simulink model "Solar_Batt_H2_PowerFlow_Solution"  (R2021a)
settings: Solver=ode8  StartTime=0.0  StopTime=8760  FixedStep=1  RelTol=1e-3
settings Model: Creator=pacel  LastModifiedBy=pacel

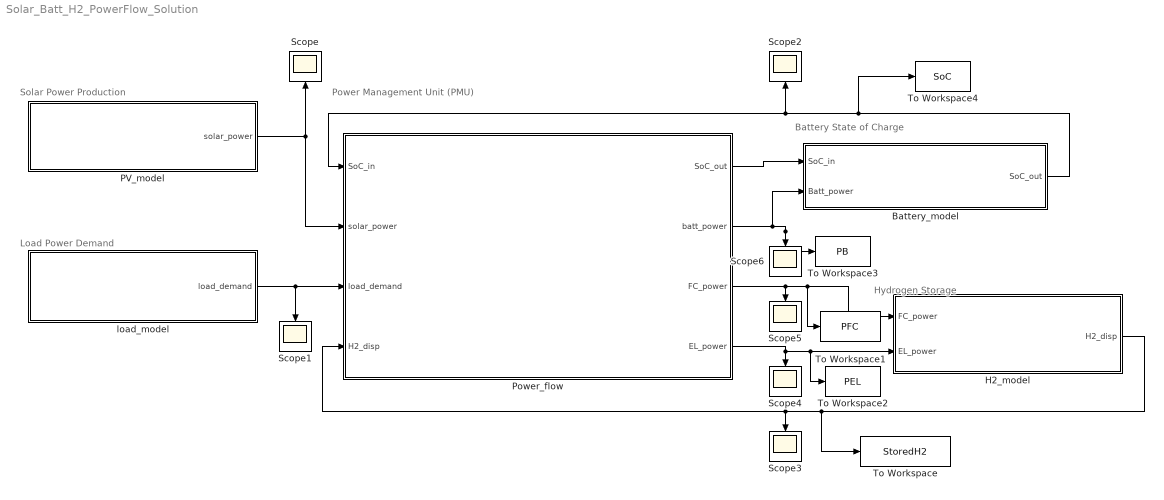
== system Solar_Batt_H2_PowerFlow_Solution ==
  note: Solar Power Production
  note: Load Power Demand
  note: Battery State of Charge
  note: Hydrogen Storage
  note: Power Management Unit (PMU)
  Battery_model : Subsystem
  H2_model : Subsystem
  PV_model : Subsystem
  Power_flow : Subsystem
  Scope{,1..6} (7 alike) : Scope
  To Workspace : ToWorkspace  VariableName=StoredH2  SaveFormat=Timeseries  SampleTime=-1
  To Workspace1 : ToWorkspace  VariableName=PFC  SaveFormat=Timeseries  SampleTime=-1
  To Workspace2 : ToWorkspace  VariableName=PEL  SaveFormat=Timeseries  SampleTime=-1
  To Workspace3 : ToWorkspace  VariableName=PB  SaveFormat=Timeseries  SampleTime=-1
  To Workspace4 : ToWorkspace  VariableName=SoC  SaveFormat=Timeseries  SampleTime=-1
  load_model : Subsystem
  wires:
  Power_flow/4(EL_power) -> Scope4/1, To Workspace2/1, H2_model/2(EL_power)
  Power_flow/3(FC_power) -> Scope5/1, H2_model/1(FC_power), To Workspace1/1
  Power_flow/2(batt_power) -> Battery_model/2(Batt_power), Scope6/1, To Workspace3/1
  H2_model/1(H2_disp) -> To Workspace/1, Power_flow/4(H2_disp), Scope3/1
  load_model/1(load_demand) -> Scope1/1, Power_flow/3(load_demand)
  PV_model/1(solar_power) -> Power_flow/2(solar_power), Scope/1
  Battery_model/1(SoC_out) -> To Workspace4/1, Scope2/1, Power_flow/1(SoC_in)
  Power_flow/1(SoC_out) -> Battery_model/1(SoC_in)

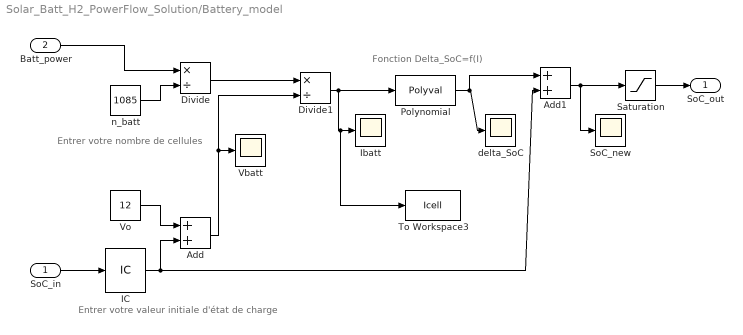
== system Solar_Batt_H2_PowerFlow_Solution/Battery_model ==
  note: Entrer votre valeur initiale d'état de charge
  note: Entrer votre nombre de cellules
  note: Fonction Delta_SoC=f(I)
  SoC_in : Inport
  Batt_power : Inport  Port=2
  Add : Sum
  Add1 : Sum
  Divide : Product  Inputs=*/
  Divide1 : Product  Inputs=*/
  IC : InitialCondition  Value=0.5
  Ibatt : Scope
  Polynomial : Polyval  Coefs=[ +8e-5, +0.0105, -0.008 ]
  Saturation : Saturate  UpperLimit=0.95  LowerLimit=0.05
  SoC_new : Scope
  To Workspace3 : ToWorkspace  VariableName=Icell  SaveFormat=Timeseries  SampleTime=-1
  Vbatt : Scope
  Vo : Constant  Value=12
  delta_SoC : Scope
  n_batt : Constant  Value=1085
  SoC_out : Outport
  wires:
  Saturation/1 -> SoC_out/1
  IC/1 -> Add1/2, Add/2
  Add1/1 -> Saturation/1, SoC_new/1
  Batt_power/1 -> Divide/1
  Add/1 -> Divide1/2, Vbatt/1
  SoC_in/1 -> IC/1
  Vo/1 -> Add/1
  Divide1/1 -> Polynomial/1, To Workspace3/1, Ibatt/1
  Divide/1 -> Divide1/1
  Polynomial/1 -> Add1/1, delta_SoC/1
  n_batt/1 -> Divide/2

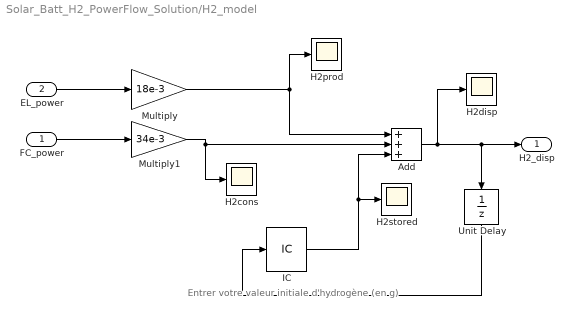
== system Solar_Batt_H2_PowerFlow_Solution/H2_model ==
  note: Entrer votre valeur initiale d'hydrogène (en g)
  FC_power : Inport
  EL_power : Inport  Port=2
  Add : Sum  Inputs=+++
  H2cons : Scope
  H2disp : Scope
  H2prod : Scope
  H2stored : Scope
  IC : InitialCondition  Value=1.2e6
  Multiply : Gain  Gain=18e-3
  Multiply1 : Gain  Gain=34e-3
  Unit Delay : UnitDelay  SampleTime=-1  HasFrameUpgradeWarning=on
  H2_disp : Outport
  wires:
  IC/1 -> Add/3, H2stored/1
  Unit Delay/1 -> IC/1
  FC_power/1 -> Multiply1/1
  EL_power/1 -> Multiply/1
  Multiply/1 -> Add/1, H2prod/1
  Multiply1/1 -> H2cons/1, Add/2
  Add/1 -> Unit Delay/1, H2_disp/1, H2disp/1

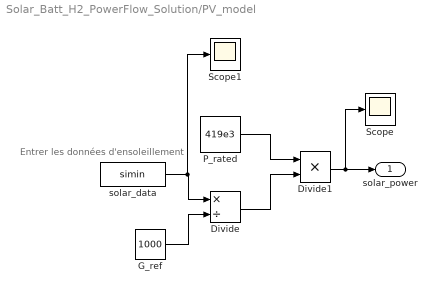
== system Solar_Batt_H2_PowerFlow_Solution/PV_model ==
  note: Entrer les données d'ensoleillement
  Divide : Product  Inputs=*/
  Divide1 : Product  Inputs=**
  G_ref : Constant  Value=1000
  P_rated : Constant  Value=419e3
  Scope : Scope
  Scope1 : Scope
  solar_data : FromWorkspace  VariableName=simin  OutDataTypeStr=double  SampleTime=1
  solar_power : Outport
  wires:
  Divide/1 -> Divide1/2
  P_rated/1 -> Divide1/1
  solar_data/1 -> Scope1/1, Divide/1
  Divide1/1 -> solar_power/1, Scope/1
  G_ref/1 -> Divide/2

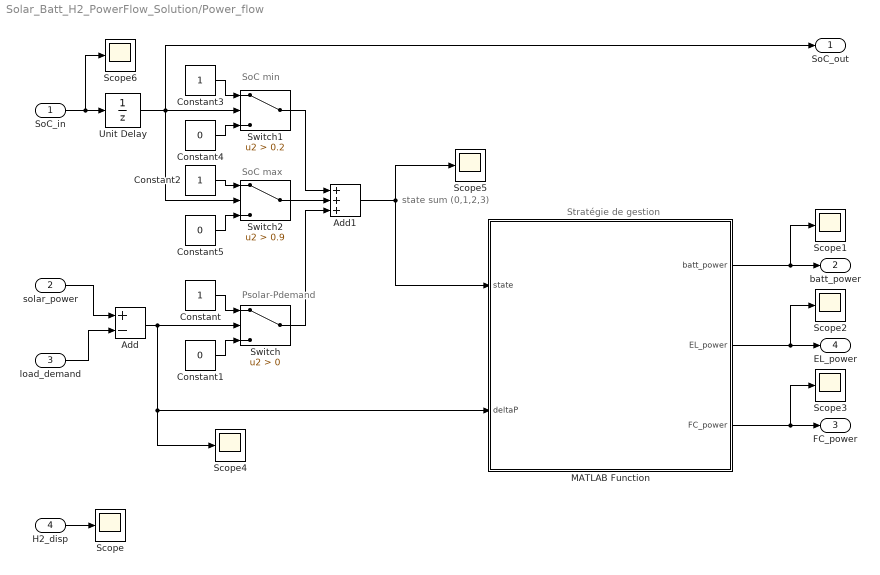
== system Solar_Batt_H2_PowerFlow_Solution/Power_flow ==
  note: SoC min
  note: SoC max
  note: Psolar-Pdemand
  note: Stratégie de gestion
  note: state sum (0,1,2,3)
  SoC_in : Inport
  solar_power : Inport  Port=2
  load_demand : Inport  Port=3
  H2_disp : Inport  Port=4
  Add : Sum  Inputs=+-
  Add1 : Sum  Inputs=+++
  Constant : Constant
  Constant1 : Constant  Value=0
  Constant2 : Constant
  Constant3 : Constant
  Constant4 : Constant  Value=0
  Constant5 : Constant  Value=0
  MATLAB Function : MATLAB Function  TreatAsAtomicUnit=on
  Scope{,1..6} (7 alike) : Scope
  Switch : Switch  Criteria=u2 > Threshold
  Switch1 : Switch  Criteria=u2 > Threshold  Threshold=0.2
  Switch2 : Switch  Criteria=u2 > Threshold  Threshold=0.9
  Unit Delay : UnitDelay  SampleTime=-1  HasFrameUpgradeWarning=on
  SoC_out : Outport
  batt_power : Outport  Port=2
  FC_power : Outport  Port=3
  EL_power : Outport  Port=4
  wires:
  H2_disp/1 -> Scope/1
  Unit Delay/1 -> SoC_out/1, Switch2/2, Switch1/2
  MATLAB Function/3(FC_power) -> FC_power/1, Scope3/1
  solar_power/1 -> Add/1
  Add1/1 -> MATLAB Function/1(state), Scope5/1
  Constant3/1 -> Switch1/1
  SoC_in/1 -> Scope6/1, Unit Delay/1
  Constant/1 -> Switch/1
  Constant1/1 -> Switch/3
  load_demand/1 -> Add/2
  Constant4/1 -> Switch1/3
  MATLAB Function/2(EL_power) -> EL_power/1, Scope2/1
  MATLAB Function/1(batt_power) -> batt_power/1, Scope1/1
  Constant2/1 -> Switch2/1
  Constant5/1 -> Switch2/3
  Switch2/1 -> Add1/2
  Add/1 -> Scope4/1, MATLAB Function/2(deltaP), Switch/2
  Switch1/1 -> Add1/1
  Switch/1 -> Add1/3

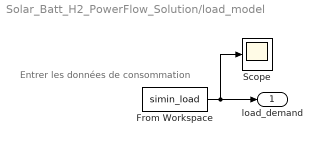
== system Solar_Batt_H2_PowerFlow_Solution/load_model ==
  note: Entrer les données de consommation
  From Workspace : FromWorkspace  VariableName=simin_load  OutDataTypeStr=double  SampleTime=1
  Scope : Scope
  load_demand : Outport
  wires:
  From Workspace/1 -> load_demand/1, Scope/1

== matlab function Solar_Batt_H2_PowerFlow_Solution/Power_flow/MATLAB Function ==
  data: state input; batt_power output; deltaP input; EL_power output; FC_power output
function [batt_power,EL_power,FC_power] = fcn(state,deltaP)
if state==0
    batt_power=0;
    EL_power=0;
    FC_power=deltaP;
elseif state==3
    batt_power=0;
    EL_power=deltaP;
    FC_power=0;
else
    batt_power=deltaP;
    EL_power=0;
    FC_power=0;
end
